simulink model "ChirpTest"  (R2021b)
settings: Solver=VariableStepAuto  StartTime=0.0  StopTime=30.0  RelTol=1e-3
libraries: simulink x1
settings Model: Creator=westwick  LastModifiedBy=randy
settings SolverCC: AlgebraicLoopSolver=TrustRegion
settings DebuggingCC: SFMachineParentedDataDiag=warning
settings SFSimCC: CustomCodeUndefinedFunction=UseInterfaceOnly

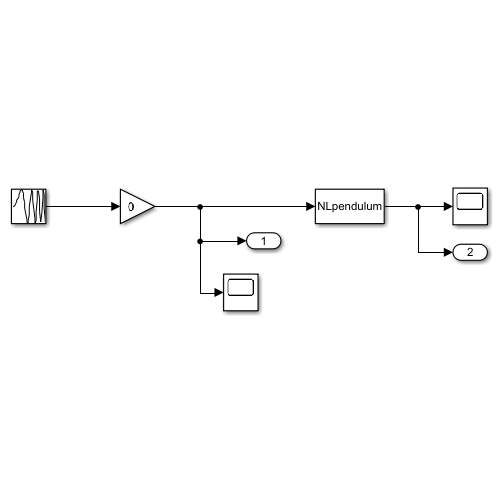
[thumbnail: Simulink's stored preview of the top-level diagram]
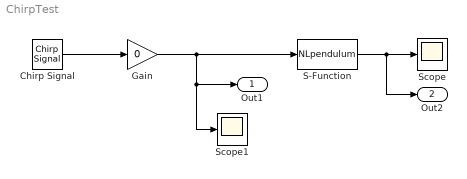
== system ChirpTest ==
  Chirp Signal : simulink/Sources/Chirp Signal  f1=0.2  T=30  f2=2
  Gain : Gain  Gain=0
  S-Function : S-Function  FunctionName=NLpendulum  SFunctionDeploymentMode=off  EnableBusSupport=off
  Scope : Scope
  Scope1 : Scope
  Out1 : Outport  VectorParamsAs1DForOutWhenUnconnected=off
  Out2 : Outport  Port=2  VectorParamsAs1DForOutWhenUnconnected=off
  wires:
  Gain/1 -> Out1/1, Scope1/1, S-Function/1
  Chirp Signal/1 -> Gain/1
  S-Function/1 -> Out2/1, Scope/1
